simulink model "gNautilus_REC_Data_Time(2015a)"  (R2015a)
settings: Solver=FixedStepDiscrete  StartTime=0.0  StopTime=180  RelTol=1e-3
model workspace (MAT data in the model file):
  cfg_native : struct (value not decoded)
  en_add_channels = 127
  host_ip = 2130706433
  host_port = 50223
  local_ip = 2130706433
  local_port = 50224
  num_en_channels = 8
  num_samples = 4
  sample_rate = 250
  serial_number = 'NB-2016.09.84'
undefined symbols (not defined in the file): NB
libraries: gNautilusLib x1, gNautilusTools x1, gtecHighspeedLib x1
settings Model: DataTypeOverride=Single  Creator=g.tec Maresch  LastModifiedBy=Gabriel
settings DataIOCC: SignalLoggingSaveFormat=ModelDataLogs
settings OptimizationCC: ExpressionDepthLimit=2147483647
settings DebuggingCC: UnderspecifiedInitializationDetection=Classic  MergeDetectMultiDrivingBlocksExec=none  SolverPrmCheckMsg=warning  FcnCallInpInsideContextMsg=EnableAllAsWarning  FrameProcessingCompatibilityMsg=none  StateNameClashWarn=warning
settings GRTTargetCC: CombineOutputUpdateFcns=off  GRTInterface=on

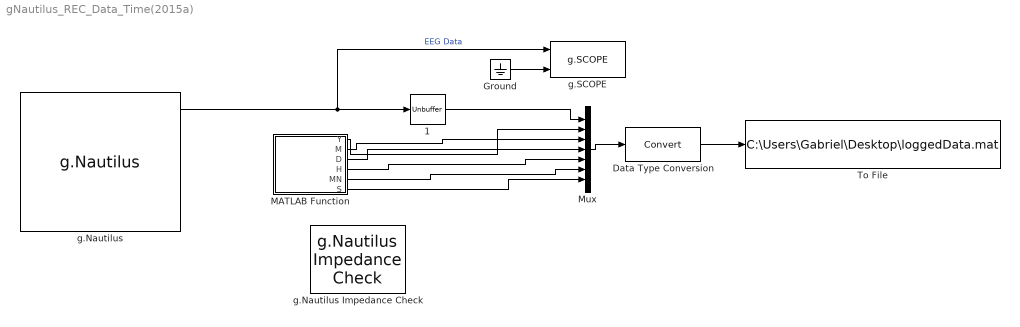
== system gNautilus_REC_Data_Time(2015a) ==
  1 : Unbuffer
  Data Type Conversion : DataTypeConversion
  Ground : Ground
  MATLAB Function : MATLAB Function  TreatAsAtomicUnit=on
      settings: PermitHierarchicalResolution=ParametersOnly
  Mux : Mux  Inputs=7
  To File : ToFile  Filename=C:\Users\Gabriel\Desktop\loggedData.mat  MatrixName=y
  g.Nautilus : gNautilusLib/g.Nautilus  Tag=g.Nautilus  Description=Operates a g.Nautilus device and provides acquired data on its outputs.  sample_rate=250  local_ip=2130706433  local_port=50224  host_ip=2130706433  host_port=50223  serial_number=NB-2016.09.84  num_samples=4  num_en_channels=8  add_channels=127
  g.Nautilus Impedance Check : gNautilusTools/g.Nautilus Impedance Check
  g.SCOPE : gtecHighspeedLib/g.SCOPE
  wires:
  g.Nautilus/1 -> g.SCOPE/1, 1/1  "EEG Data"
  Data Type Conversion/1 -> To File/1
  Mux/1 -> Data Type Conversion/1
  1/1 -> Mux/1
  Ground/1 -> g.SCOPE/2
  MATLAB Function/5(MN) -> Mux/6
  MATLAB Function/4(H) -> Mux/5
  MATLAB Function/3(D) -> Mux/4
  MATLAB Function/1(Y) -> Mux/2
  MATLAB Function/2(M) -> Mux/3
  MATLAB Function/6(S) -> Mux/7

== matlab function gNautilus_REC_Data_Time(2015a)/MATLAB Function ==
  data: Y output; M output; D output; H output; MN output; S output
function [Y, M, D, H, MN, S] = fcn()
   coder.extrinsic('now');
   coder.extrinsic('datevec');
   Y = 0;
   M = 0;
   D = 0;
   H = 0;
   MN = 0;
   S = 0;
   [Y, M, D, H, MN, S] = datevec(now);
end
